simulink model "syn_weight_trace_elig_single_synapse"  (R2024a)
settings: Solver=VariableStepAuto  StartTime=0.0  StopTime=4.0  RelTol=1e-3
values from neighbouring files (symbols this model uses):
  eta_d = 200    [synaptic_weight_ode45.m]
  eta_p = 0.2    [synaptic_weight_ode45.m]
  tau_d = 1.5    [synaptic_weight_ode45.m]
  tau_p = 0.2    [synaptic_weight_ode45.m]
  Tmax_d = 2    [synaptic_weight_ode45.m]
  Tmax_p = 2.2    [synaptic_weight_ode45.m]
settings Model: Creator=Aleksandar Kežić  LastModifiedBy=Aleksandar Kežić

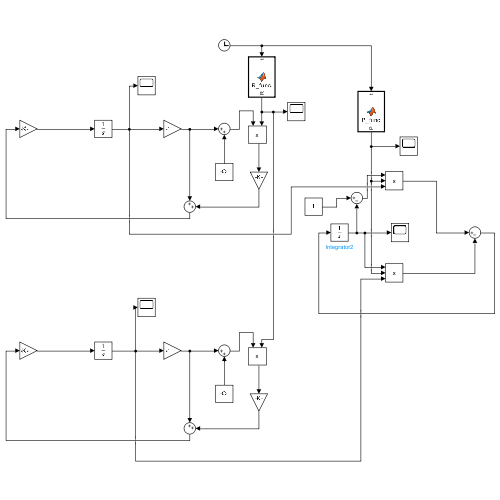
[thumbnail: Simulink's stored preview of the top-level diagram]
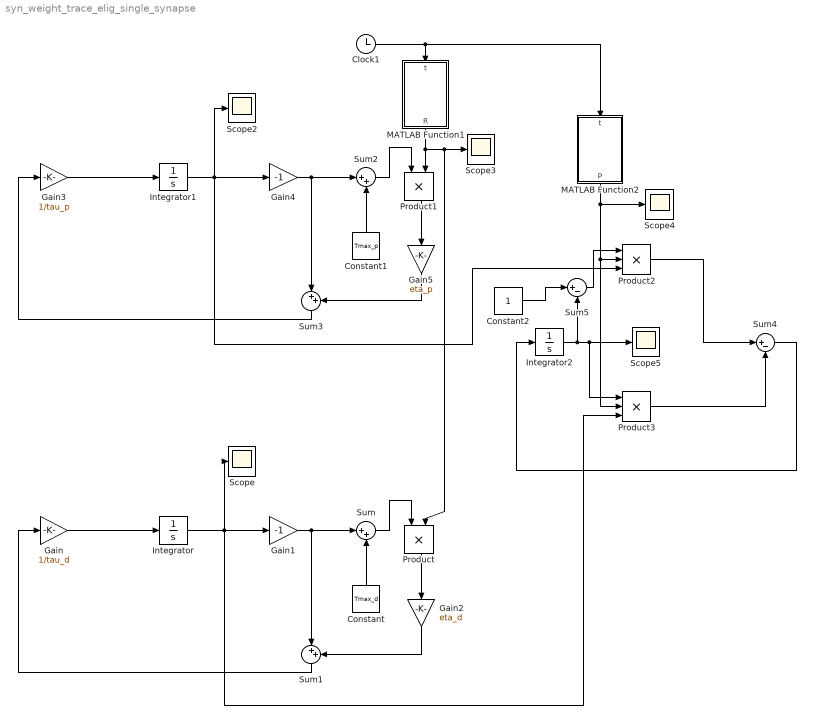
== system syn_weight_trace_elig_single_synapse ==
  Clock1 : Clock
  Constant : Constant  Value=Tmax_d
  Constant1 : Constant  Value=Tmax_p
  Constant2 : Constant
  Gain : Gain  Gain=1/tau_d
  Gain1 : Gain  Gain=-1
  Gain2 : Gain  Gain=eta_d
  Gain3 : Gain  Gain=1/tau_p
  Gain4 : Gain  Gain=-1
  Gain5 : Gain  Gain=eta_p
  Integrator : Integrator
  Integrator1 : Integrator
  Integrator2 : Integrator
  MATLAB Function1 : MATLAB Function  TreatAsAtomicUnit=on
  MATLAB Function2 : MATLAB Function  TreatAsAtomicUnit=on
  Product : Product
  Product1 : Product
  Product2 : Product  Inputs=3
  Product3 : Product  Inputs=3
  Scope{,2..5} (5 alike) : Scope
  Sum{,1..3} (4 alike) : Sum  Inputs=|++
  Sum4 : Sum  Inputs=|+-
  Sum5 : Sum  Inputs=|+-
  wires:
  Gain/1 -> Integrator/1
  Integrator/1 -> Scope/1, Product3/3, Gain1/1
  Gain1/1 -> Sum/1, Sum1/1
  Gain2/1 -> Sum1/2
  Constant/1 -> Sum/2
  Product/1 -> Gain2/1
  Sum/1 -> Product/1
  Sum1/1 -> Gain/1
  Gain4/1 -> Sum2/1, Sum3/1
  Sum2/1 -> Product1/1
  Gain5/1 -> Sum3/2
  Constant1/1 -> Sum2/2
  Gain3/1 -> Integrator1/1
  Integrator1/1 -> Product2/3, Scope2/1, Gain4/1
  Product1/1 -> Gain5/1
  Clock1/1 -> MATLAB Function2/1(t), MATLAB Function1/1(t)
  MATLAB Function1/1(R) -> Product/2, Scope3/1, Product1/2
  Sum3/1 -> Gain3/1
  Integrator2/1 -> Scope5/1, Product3/1, Sum5/2
  Product3/1 -> Sum4/2
  Product2/1 -> Sum4/1
  Sum4/1 -> Integrator2/1
  MATLAB Function2/1(P) -> Scope4/1, Product3/2, Product2/2
  Sum5/1 -> Product2/1
  Constant2/1 -> Sum5/1

== matlab function syn_weight_trace_elig_single_synapse/MATLAB Function2 ==
  data: t input; P output
function P = P_func(t)
    gamma = 1.0;
    tau_I = 3.5;
    tP = 0.6;
    if t < tP
        P = 0;
    else
        P = gamma * exp(-(t - tP)/tau_I);
    end
end

== matlab function syn_weight_trace_elig_single_synapse/MATLAB Function1 ==
  data: t input; R output
function R = R_func(t)
    alpha = 7.5;
    sigma = 0.9/(3*sqrt(2));
    v = 0.5;
    x0 = 0.4; % place field center of a single synapse
    R = alpha * exp(-((v*t - x0)/sigma)^2);
end
